simulink model "two_MSD_system"  (R2023a)
settings: Solver=FixedStepAuto  StartTime=0.0  StopTime=300.0  RelTol=1e-3
undefined symbols (not defined in the file): b1, b2, k1, k2, m1, m2
settings Model: Creator=kaiad  LastModifiedBy=kaiad

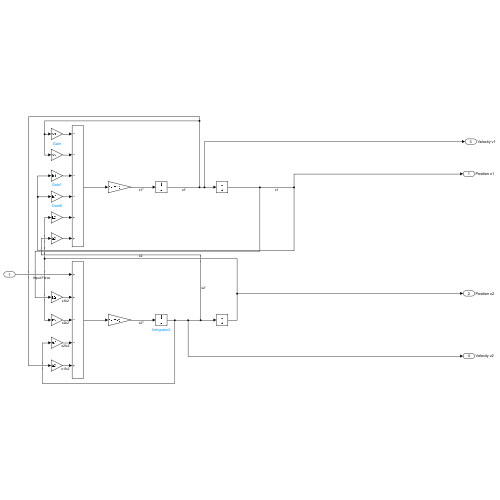
[thumbnail: Simulink's stored preview of the top-level diagram]
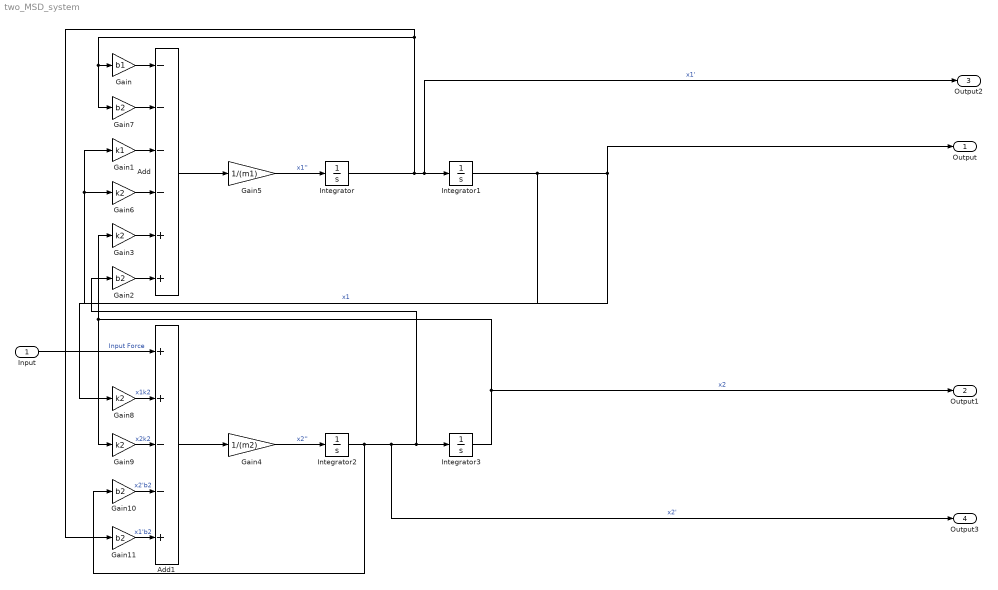
== system two_MSD_system ==
  Input : Inport
  Add : Sum  Inputs=----++
  Add1 : Sum  Inputs=++--+
  Gain : Gain  Gain=b1
  Gain1 : Gain  Gain=k1
  Gain{2,7,10..11} (4 alike) : Gain  Gain=b2
  Gain{3,6,8..9} (4 alike) : Gain  Gain=k2
  Gain4 : Gain  Gain=1/(m2)
  Gain5 : Gain  Gain=1/(m1)
  Integrator : Integrator
  Integrator1 : Integrator  InitialCondition=5
  Integrator2 : Integrator
  Integrator3 : Integrator  InitialCondition=7
  Output : Outport  SignalName=Position x1
  Output1 : Outport  Port=2  SignalName=Position x2
  Output2 : Outport  Port=3  SignalName=Velocity v1
  Output3 : Outport  Port=4  SignalName=Velocity v2
  wires:
  Integrator/1 -> Gain7/1, Gain/1, Gain11/1, Output2/1, Integrator1/1  "x1'"
  Integrator2/1 -> Output3/1, Gain2/1, Integrator3/1, Gain10/1  "x2'"
  Integrator1/1 -> Gain8/1, Gain1/1, Gain6/1, Output/1  "x1"
  Integrator3/1 -> Gain3/1, Gain9/1, Output1/1  "x2"
  Gain4/1 -> Integrator2/1  "x2''"
  Gain5/1 -> Integrator/1  "x1''"
  Add/1 -> Gain5/1
  Gain3/1 -> Add/5
  Gain2/1 -> Add/6
  Gain6/1 -> Add/4
  Gain1/1 -> Add/3
  Gain7/1 -> Add/2
  Gain/1 -> Add/1
  Gain11/1 -> Add1/5  "x1'b2"
  Gain9/1 -> Add1/3  "x2k2"
  Gain10/1 -> Add1/4  "x2'b2"
  Gain8/1 -> Add1/2  "x1k2"
  Input/1 -> Add1/1  "Input Force"
  Add1/1 -> Gain4/1
